simulink model "LQR_min_obs_noise"  (R2025b)
settings: Solver=VariableStepAuto  StartTime=0.0  StopTime=100  RelTol=1e-3
values from neighbouring files (symbols this model uses):
  a = -log(OS/100)    [pole_placement_ctrl.m]
  A = [0 1 0 0;     (m_b*g*r^2)/(I_b*l) 0 (m_b*g*r^2)/(I_b) 0 ;      0 0 0 1;    20 0 (M_r*d*g)/I_r 0 ]    [Copy_of_LQR_ctrl.m]    (also in LQR_ctrl.m = [0 1 0 0;     A1(1,1) 0 A1(1,2) 0;     0 0 0 1;     A1(2,1) ; Rlocus_ctrl.m = [0 1 0 0;     A1(1,1) 0 A1(1,2) 0;     0 0 0 1;     A1(2,1) ; State4.m = [0 1 0 0;     A1(1,1) 0 A1(1,2) 0;     0 0 0 1;     A1(2,1) ; pole_placement_ctrl.m = [0 1 0 0;     A1(1,1) 0 A1(1,2) 0;     0 0 0 1;     A1(2,1) )
  A_hat = A_bb - Ke_min*A_ab    [Copy_of_LQR_ctrl.m]    (also in LQR_ctrl.m)
  B = -[0 ; 0; 0 ; ((I_w/R) + (M_w+M_r)*R)/(I_r)]    [Copy_of_LQR_ctrl.m]    (also in LQR_ctrl.m = -[0 ; B1(1); 0 ; B1(2)]; Rlocus_ctrl.m = -[0 ; B1(1); 0 ; B1(2)]; State4.m = -[0 ; B1(1); 0 ; B1(2)]; pole_placement_ctrl.m = -[0 ; B1(1); 0 ; B1(2)])
  B_hat = A_hat*Ke_min + A_ba - Ke_min*A_aa    [Copy_of_LQR_ctrl.m]    (also in LQR_ctrl.m)
  C = [0 0 1 0]    [Copy_of_LQR_ctrl.m]    (also in LQR_ctrl.m; Rlocus_ctrl.m = eye(4); State4.m = eye(4); pole_placement_ctrl.m = eye(4))
  C_hat = zeros(4, nb)    [Copy_of_LQR_ctrl.m]    (also in LQR_ctrl.m)
  D_hat = zeros(4, na)    [Copy_of_LQR_ctrl.m]    (also in LQR_ctrl.m)
  F_hat = B_b - Ke_min*B_a    [Copy_of_LQR_ctrl.m]    (also in LQR_ctrl.m)
  K = lqr(A, B, Q, R)    [State4.m]    (also in pole_placement_ctrl.m = place(A,B,poles))
  x0 = [0.01, 0, deg2rad(5),0]'    [Copy_of_LQR_ctrl.m]    (also in LQR_ctrl.m; State4.m = x0 - x_ref; pole_placement_ctrl.m = [0.005;0;deg2rad(0);0])
  x0_omin = [-0.002;0;0]    [Copy_of_LQR_ctrl.m]    (also in LQR_ctrl.m = [-0.02;0;0])
undefined symbols (not defined in the file or in its folder): b, dspblkCoreblockFVToolHelper, gcbh
libraries: simulink x1
settings Model: Creator=Abhi  LastModifiedBy=Abhi

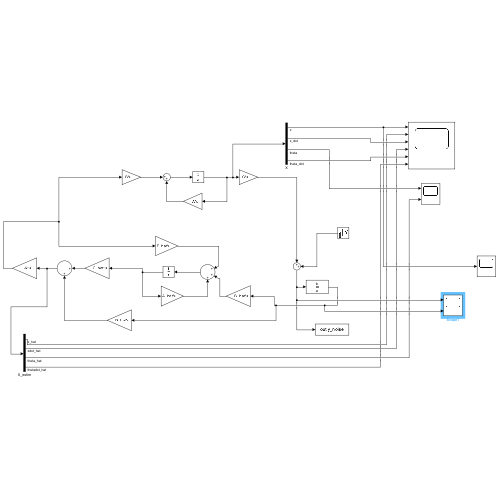
[thumbnail: Simulink's stored preview of the top-level diagram]
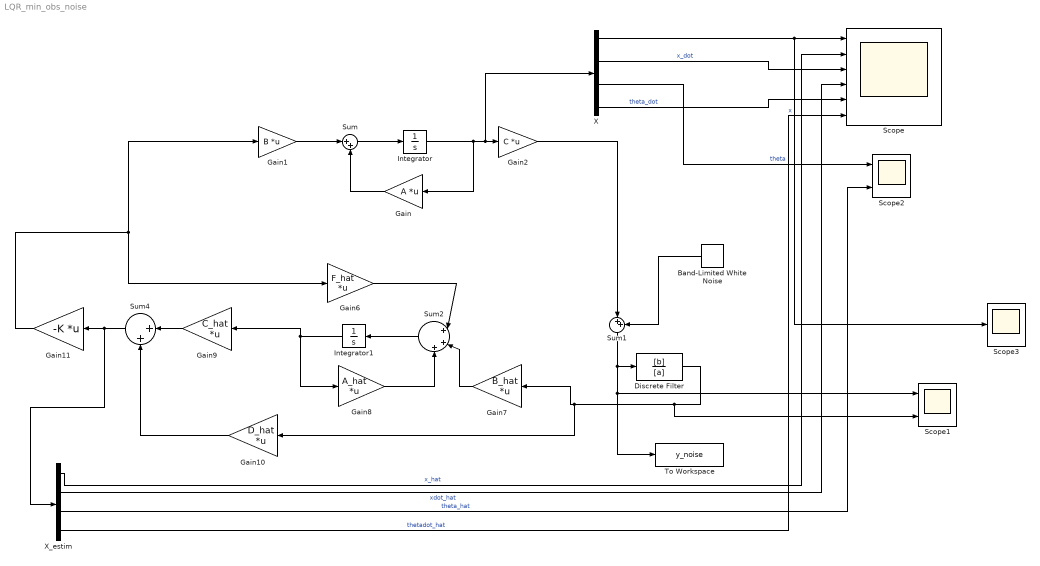
== system LQR_min_obs_noise ==
  Band-Limited White Noise : simulink/Sources/Band-Limited White Noise  Cov=0.00000000005  Ts=1e-4  seed=[23341]
  Discrete Filter : DiscreteFilter  LoadFcn=dspblkCoreblockFVToolHelper(gcbh,'load');  Numerator=[b]  Denominator=[a]
      settings: CopyFcn=dspblkCoreblockFVToolHelper(gcbh,'copy');  DeleteFcn=dspblkCoreblockFVToolHelper(gcbh,'close');  ModelCloseFcn=dspblkCoreblockFVToolHelper(gcbh,'close');  PreSaveFcn=dspblkCoreblockFVToolHelper(gcbh,'presave');  PostSaveFcn=dspblkCoreblockFVToolHelper(gcbh,'postsave');  CloseFcn=dspblkCoreblockFVToolHelper(gcbh,'close');
  Gain : Gain  Gain=A  Multiplication=Matrix(K*u)
  Gain1 : Gain  Gain=B  Multiplication=Matrix(K*u)
  Gain10 : Gain  Gain=D_hat  Multiplication=Matrix(K*u)
  Gain11 : Gain  Gain=-K  Multiplication=Matrix(K*u)
  Gain2 : Gain  Gain=C  Multiplication=Matrix(K*u)
  Gain6 : Gain  Gain=F_hat  Multiplication=Matrix(K*u)
  Gain7 : Gain  Gain=B_hat  Multiplication=Matrix(K*u)
  Gain8 : Gain  Gain=A_hat  Multiplication=Matrix(K*u)
  Gain9 : Gain  Gain=C_hat  Multiplication=Matrix(K*u)
  Integrator : Integrator  InitialCondition=x0
  Integrator1 : Integrator  InitialCondition=x0_omin
  Scope : Scope  NumInputPorts=6
      settings: SampleTime=1e-4  ActiveDisplayYMinimum=-0.037800906184902339  ActiveDisplayYMaximum=0.055197898912851991
  Scope1 : Scope  NumInputPorts=2
      settings: SampleTime=1e-4  ActiveDisplayYMinimum=-0.017776250388577511  ActiveDisplayYMaximum=0.10132926804150635
  Scope2 : Scope  NumInputPorts=2
      settings: SampleTime=1e-4  ActiveDisplayYMinimum=-0.041102850477065939  ActiveDisplayYMaximum=0.020859803894727538  DataLoggingVariableName=ScopeData2
  Scope3 : Scope
      settings: SampleTime=1e-4  ActiveDisplayYMinimum=-0.03764065399801178  ActiveDisplayYMaximum=0.055219942526110913  DataLoggingVariableName=ScopeData3
  Sum : Sum  Inputs=|++
  Sum1 : Sum  Inputs=|++
  Sum2 : Sum  Inputs=|+++
  Sum4 : Sum  Inputs=|++
  To Workspace : ToWorkspace  VariableName=y_noise  SaveFormat=Structure With Time  SampleTime=1e-4
  X : Demux
  X_estim : Demux
  wires:
  Sum/1 -> Integrator/1
  Sum4/1 -> X_estim/1, Gain11/1
  X/3 -> Scope2/1  "theta"
  Integrator1/1 -> Gain9/1, Gain8/1
  X_estim/1 -> Scope/2  "x_hat"
  X_estim/3 -> Scope2/2  "theta_hat"
  Integrator/1 -> X/1, Gain2/1, Gain/1
  X_estim/2 -> Scope/4  "xdot_hat"
  Gain11/1 -> Gain1/1, Gain6/1
  X_estim/4 -> Scope/6  "thetadot_hat"
  Gain7/1 -> Sum2/2
  Gain9/1 -> Sum4/1
  X/2 -> Scope/3  "x_dot"
  X/1 -> Scope3/1, Scope/1  "x"
  Gain8/1 -> Sum2/3
  Gain10/1 -> Sum4/2
  Gain/1 -> Sum/2
  Gain6/1 -> Sum2/1
  X/4 -> Scope/5  "theta_dot"
  Gain1/1 -> Sum/1
  Sum2/1 -> Integrator1/1
  Band-Limited White Noise/1 -> Sum1/2
  Gain2/1 -> Sum1/1
  Sum1/1 -> Scope1/1, To Workspace/1, Discrete Filter/1
  Discrete Filter/1 -> Scope1/2, Gain10/1, Gain7/1
